simulink model "KinControl_DELTA"  (R2018b)
settings: Solver=FixedStepAuto  StartTime=0.0  StopTime=10  FixedStep=0.001  RelTol=1e-5
model workspace (MAT data in the model file):
  I_bc = 0.466666666667
  I_bi = 2.46666666667
  I_brake = 1
  I_m = 1
  R = 0.63
  b = 2
  ee = [0; 0; -2.1944]
  k_r = 1
  l_A = 1
  l_B = 2
  m_b = 1
  m_br = 1.13333333333
  m_c = 0
  m_fb = 0.2
  m_n = 1
  m_nt = 3.6
  m_p = 0
  r_Gb = 0.558823529412
  r_l = 0.63
  r_m = 0.666666666667
  theta = [0 2.09439510239 4.18879020479]
settings Model: Creator=enrico  LastModifiedBy=enrico

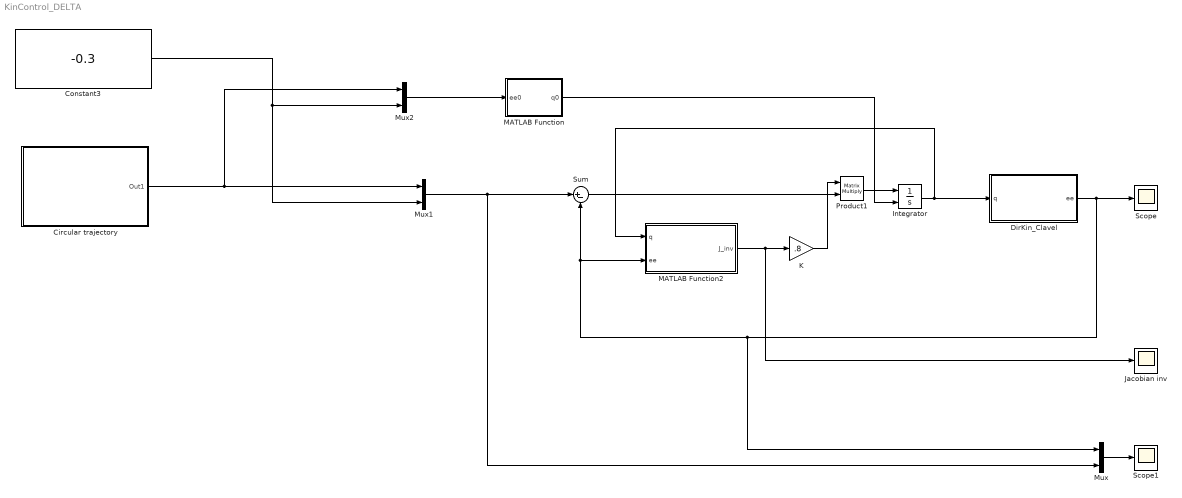
== system KinControl_DELTA ==
  Circular trajectory : Subsystem  mask{A=0.05, F=1}
      mask prompts: A "Amplitude"; F "Frequency"
  Constant3 : Constant  Value=-0.3  SampleTime=-1
  DirKin_Clavel : MATLAB Function  TreatAsAtomicUnit=on
      mask init:
      | loadvar
  Integrator : Integrator  InitialConditionSource=external
  Jacobian inv : Scope
  K : Gain  Gain=.8
  MATLAB Function : MATLAB Function  TreatAsAtomicUnit=on
  MATLAB Function2 : MATLAB Function  TreatAsAtomicUnit=on
  Mux : Mux  Inputs=2
  Mux1 : Mux  Inputs=2
  Mux2 : Mux  Inputs=2
  Product1 : Product  Multiplication=Matrix(*)
  Scope : Scope
  Scope1 : Scope
  Sum : Sum  Inputs=|+-
  wires:
  K/1 -> Product1/1
  Product1/1 -> Integrator/1
  Sum/1 -> Product1/2
  Mux2/1 -> MATLAB Function/1(ee0)
  DirKin_Clavel/1(ee) -> Scope/1, Mux/1, Sum/2, MATLAB Function2/2(ee)
  Circular trajectory/1(Out1) -> Mux2/1, Mux1/1
  Constant3/1 -> Mux1/2, Mux2/2
  MATLAB Function/1(q0) -> Integrator/2
  Mux1/1 -> Mux/2, Sum/1
  MATLAB Function2/1(J_inv) -> Jacobian inv/1, K/1
  Mux/1 -> Scope1/1
  Integrator/1 -> DirKin_Clavel/1(q), MATLAB Function2/1(q)

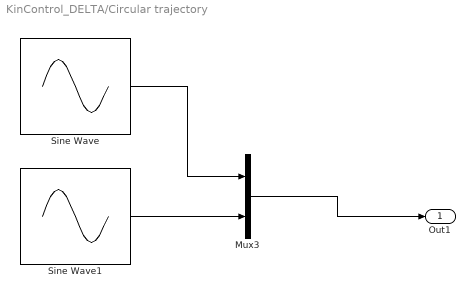
== system KinControl_DELTA/Circular trajectory ==
  Mux3 : Mux  Inputs=2
  Sine Wave : Sin  Amplitude=A  Frequency=F  Phase=pi/2
  Sine Wave1 : Sin  Amplitude=A  Frequency=F
  Out1 : Outport
  wires:
  Mux3/1 -> Out1/1
  Sine Wave/1 -> Mux3/1
  Sine Wave1/1 -> Mux3/2

== matlab function KinControl_DELTA/DirKin_Clavel ==
  data: q input; ee output
function ee = DirKin_Clavel(q)

[theta, R, ~, ~, l_A, ~, ~, l_B, ~, ~, ~] = Parameters_DELTA;

D = nan(3,1);
E = nan(3,1);
F = nan(3,1);
G = nan(3,1);

for i = 1:3
   D(i) = -l_B^2 + l_A^2 + R^2 + 2*R*l_A*cos(q(i));
   
   E(i) = 2*(R + l_A*cos(q(i)))*cos(theta(i));
   
   F(i) = 2*(R + l_A*cos(q(i)))*sin(theta(i));
   
   G(i) = -2*l_A*sin(q(i)); 
end

H = [E(1)*G(2) - E(1)*G(3) - E(2)*G(1) + E(2)*G(3) + E(3)*G(1) - E(3)*G(2);
    -E(1)*F(2) + E(1)*F(3) + E(2)*F(1) - E(2)*F(3) - E(3)*F(1) + E(3)*F(2);
    -E(1)*D(2) + E(1)*D(3) + E(2)*D(1) - E(2)*D(3) - E(3)*D(1) + E(3)*D(2);
     F(1)*D(2) - F(1)*D(3) - F(2)*D(1) + F(2)*D(3) + F(3)*D(1) - F(3)*D(2);
    -F(1)*G(2) + F(1)*G(3) + F(2)*G(1) - F(2)*G(3) - F(3)*G(1) + F(3)*G(2)];

L = (H(5)^2 + H(1)^2)/H(2)^2 + 1;

M = 2*(H(5)*H(4) + H(1)*H(3))/H(2)^2 - (H(5)*E(1) + H(1)*F(1))/H(2) - G(1);

N = (H(4)^2 + H(3)^2)/H(2)^2 - (H(4)*E(1) + H(3)*F(1))/H(2) + D(1);

ee = nan(3,1);
ee2 = nan(3,1);

ee(3) = (-M + sqrt(M^2 - 4*L*N))/(2*L);

ee(1) = ee(3)*H(5)/H(2) + H(4)/H(2);

ee(2) = ee(3)*H(1)/H(2) + H(3)/H(2);

ee2(3) = (-M - sqrt(M^2 - 4*L*N))/(2*L);

ee2(1) = ee2(3)*H(5)/H(2) + H(4)/H(2);

ee2(2) = ee2(3)*H(1)/H(2) + H(3)/H(2);
 


% if ee2(3) < 0 
%     ee = ee2;
% end

if ee(3) > ee2(3)
    ee = ee2;
end

end

== matlab function KinControl_DELTA/MATLAB Function ==
  data: ee0 input; q0 output
function q0 = InverseKinematic(ee0)
%Computation of the inverse kinematic of the Delta robot

% Loading parameters
[theta, R, ~, ~, l_A, ~, ~, l_B, ~, ~, ~] = Parameters_DELTA;

R_b1 = R_base(theta(1));
R_b2 = R_base(theta(2));
R_b3 = R_base(theta(3));
p = [R_b1\ee0, R_b2\ee0, R_b3\ee0]; 
q0 = nan(3,1);

for li=1:3
    
    x0 = p(1,li);
    y0 = p(2,li);
    z0 = p(3,li);
    A = l_A^2 - l_B^2 - R^2 + x0^2 + y0^2 + z0^2;
    B = 2*x0 - 2*R;

    a = 4*z0^2 + B^2;
    b = 4*R*z0^2 + A*B;
    c = A^2 + 4*R^2*z0^2 - 4*l_A^2*z0^2;
        
    x = (b + sqrt(b^2 - a*c))/a; 
    
    z = (A - B*x)/(2*z0);
    
    q0(li) = - asin(z/l_A); 
    
    if x-R < 0
        q0(li) = pi - q0(li);
    end    
end

end

== matlab function KinControl_DELTA/MATLAB Function2 ==
  data: q input; ee input; J_inv output
function J_inv = inv_Jacobian(q, ee)
% Give back Jacobian matrix and its derivative

[theta, R, ~, ~, l_A, ~, ~, ~, ~, ~, ~] = Parameters_DELTA;

% Initialize matrices
S = nan(3);
B = nan(3);
dB = nan(3);
dS = nan(3);

for i=1:3
    % Rotation matrix from base plate frame to i-joint frame 
    R_b = R_base(theta(i));
    
    % Matrix with s_i vectors as columns
    S(:,i) = ee - R_b*([R 0 0]' - l_A*[cos(q(i)), 0, sin(q(i))]');
    
    % Matrix with b_i vectors as columns
    B(:,i) = R_b*l_A*[-sin(q(i)), 0, cos(q(i))]';
    
    % Matrix with db_i vectors as columns
    dB(:,i) = R_b*l_A*[-cos(q(i)); 0; -sin(q(i))];
    
    % Matrix with ds_i vectors as columns
    dS(:,i) = ee - R_b*l_A*[-sin(q(i)), 0, cos(q(i))]';
end

% Jacobian
J = S'\diag(diag(S'*B));

J_inv = inv(J);

% J_inv = pinv(J);
end
